simulink model "Controlador_Otimo_Aerosimples"  (R2018a)
settings: Solver=FixedStepAuto  StartTime=0.0  StopTime=inf  RelTol=1e-3  EnableMultiTasking=on
values from neighbouring files (symbols this model uses):
  C = [1 0 0 0 ... (first row only)    [Dados.m]    (also in Dados_correct.m; Function_ARE.m = D; teste.m = D)
  K1 = Kpi(:,1:4)    [Dados.m]    (also in Dados_correct.m = Kpi90(:,1:4); Function_ARE.m = K(:,1:4); teste.m = K(:,1:4))
  K2 = Kpi(:,5:6)    [Dados.m]    (also in Dados_correct.m = Kpi90(:,5:6); Function_ARE.m = K(:,5:6); teste.m = K(:,5:6))
undefined symbols (not defined in the file or in its folder): DiscIntNeverNeededParam
libraries: arduinolib x2, simulink x1
settings Model: SimulationMode=external  ExtModeTrigDuration=2  Creator=stayn  LastModifiedBy=stayn
settings SolverCC: AutoInsertRateTranBlk=on
settings OptimizationCC: EnhancedBackFolding=on  PassReuseOutputArgsAs=Individual arguments  MaxStackSize=64  OptimizeBlockOrder=speed  DifferentSizesBufferReuse=on  OptimizationCustomize=off
settings DebuggingCC: ParameterTunabilityLossMsg=error
settings HardwareCC: ProdBitPerInt=16  ProdBitPerPointer=16  ProdBitPerSizeT=16  ProdBitPerPtrDiffT=16  ProdLargestAtomicFloat=None  ProdWordSize=8  ProdHWDeviceType=Atmel->AVR
settings SFSimCC: MATLABDynamicMemAlloc=off
settings RTWCC: SystemTargetFile=ert.tlc  HardwareBoard=Arduino Uno  TLCOptions=-aInlineSetEventsForThisBaseRateFcn=TLC_FALSE -aSuppressMultiTaskScheduler=TLC_FALSE -aRateBasedStepFcn=1  TemplateMakefile=ert_default_tmf  GenerateReport=on  Toolchain=Arduino AVR  BuildConfiguration=Faster Runs  IncludeHyperlinkInReport=on  LaunchReport=on  GenerateTraceInfo=on  GenerateTraceReport=on  GenerateTraceReportSl=on  GenerateTraceReportSf=on  GenerateTraceReportEml=on
settings CodeAppCC: ForceParamTrailComments=on  IgnoreCustomStorageClasses=off  OperatorAnnotations=on  SimulinkDataObjDesc=on  SFDataObjDesc=on  InsertBlockDesc=on
settings ERTTargetCC: SupportContinuousTime=on  SupportVariableSizeSignals=on

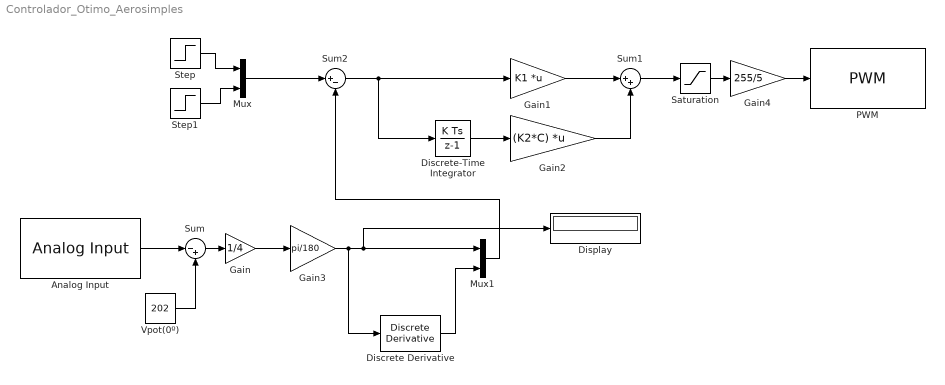
== system Controlador_Otimo_Aerosimples ==
  Analog Input : arduinolib/Analog Input  pinNumber=0  ReadResultsOnly=off  ConversionTriggerSource=Software  ExternalTriggerType=uint32(0)  OutputDataType=uint16  EnableConversionCompleteNotify=off  EnableOuputStatus=off  SampleTime=0.002  blockPlatform=arduino
  Discrete Derivative : simulink/Discrete/Discrete Derivative  gainval=1.0  ICPrevScaledInput=0.0  OutMin=[]  OutMax=[]  OutDataType=fixdt(1, 16)  OutScaling=2^-10  DoSatur=off
  Discrete-Time Integrator : DiscreteIntegrator  SampleTime=0.002  ICPrevOutput=DiscIntNeverNeededParam  ICPrevScaledInput=DiscIntNeverNeededParam
  Display : Display
  Gain : Gain  Gain=1/4
  Gain1 : Gain  Gain=K1  Multiplication=Matrix(K*u) (u vector)
  Gain2 : Gain  Gain=(K2*C)  Multiplication=Matrix(K*u) (u vector)
  Gain3 : Gain  Gain=pi/180
  Gain4 : Gain  Gain=255/5
  Mux : Mux  Inputs=2
  Mux1 : Mux  Inputs=2
  PWM : arduinolib/PWM  pinNumber=9  EnableInputFrequency=off  InitialFrequency=2000  InitialDutyCycle=0  NotificationType=None  blockPlatform=arduino
  Saturation : Saturate  UpperLimit=5  LowerLimit=0
  Step : Step  After=-0.2  SampleTime=0
  Step1 : Step  After=0  SampleTime=0
  Sum : Sum  Inputs=|-+
  Sum1 : Sum  Inputs=|++
  Sum2 : Sum  Inputs=|+-
  Vpot(0º) : Constant  Value=202
  wires:
  Analog Input/1 -> Sum/1
  Sum/1 -> Gain/1
  Vpot(0º)/1 -> Sum/2
  Gain/1 -> Gain3/1
  Step/1 -> Mux/1
  Step1/1 -> Mux/2
  Mux/1 -> Sum2/1
  Gain2/1 -> Sum1/2
  Discrete-Time Integrator/1 -> Gain2/1
  Gain1/1 -> Sum1/1
  Sum2/1 -> Discrete-Time Integrator/1, Gain1/1
  Sum1/1 -> Saturation/1
  Saturation/1 -> Gain4/1
  Discrete Derivative/1 -> Mux1/2
  Mux1/1 -> Sum2/2
  Gain3/1 -> Discrete Derivative/1, Display/1, Mux1/1
  Gain4/1 -> PWM/1
